simulink model "model"  (Simulink 8.7)
settings: Solver=VariableStepAuto  SolverMode=SingleTasking  StartTime=0.0  StopTime=10.0  RelTol=1e-3
settings Model: Creator=Kostyaj  LastModifiedBy=morozov
settings DataIOCC: LimitDataPoints=off  SaveFormat=Dataset
settings DebuggingCC: UnderspecifiedInitializationDetection=Simplified  MergeDetectMultiDrivingBlocksExec=error  SFUnexpectedBacktrackingDiag=error  SFNoUnconditionalDefaultTransitionDiag=error
settings HardwareCC: ProdBitPerPointer=64  ProdLargestAtomicFloat=Float  ProdIntDivRoundTo=Zero  ProdEndianess=LittleEndian  ProdWordSize=64  ProdHWDeviceType=Intel->x86-64 (Windows64)
settings ModelReferenceCC: PropagateSignalLabelsOutOfModel=on
settings GRTTargetCC: TargetLangStandard=C99 (ISO)  GeneratePreprocessorConditionals=Use local settings
settings ConfigComp: CovMetricSettings=dwe  CovHtmlReporting=off  CovSaveCumulativeToWorkspaceVar=off  CovSaveSingleToWorkspaceVar=off  CovModelRefEnable=off  CovExternalEMLEnable=on

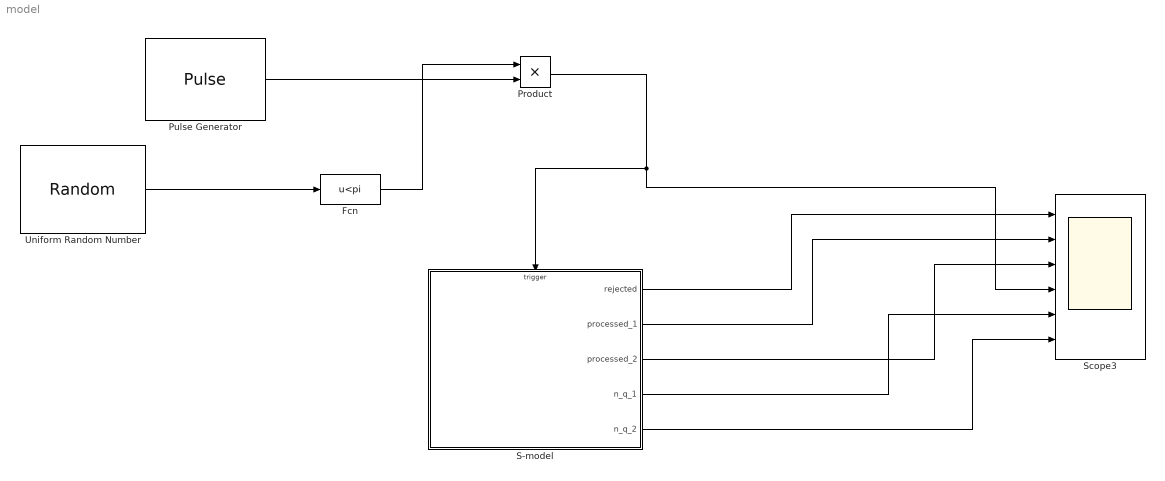
== system model ==
  Fcn : Fcn  Expr=u<pi
  Product : Product
  Pulse Generator : DiscretePulseGenerator  PulseType=Time based  Period=10  PulseWidth=5
  "S-model " : Stateflow chart  TreatAsAtomicUnit=on
  Scope3 : Scope  NumInputPorts=6
  Uniform Random Number : UniformRandomNumber  SampleTime=0.1
  wires:
  Uniform Random Number/1 -> Fcn/1
  Fcn/1 -> Product/1
  Pulse Generator/1 -> Product/2
  Product/1 -> "S-model "/Trigger, Scope3/4
  "S-model "/1(rejected) -> Scope3/1
  "S-model "/2(processed_1) -> Scope3/2
  "S-model "/3(processed_2) -> Scope3/3
  "S-model "/4(n_q_1) -> Scope3/5
  "S-model "/5(n_q_2) -> Scope3/6

== stateflow chart S-model  ==
  settings: sampleTime=Ts
  state Generator [parallel]
    settings: executionOrder=1
    state free/
    (junction 23) -> Generator.free [order 2] : [in(Q1.Process.free)]
        | {send(query, Q1.Process);}
    (junction 23) -> Generator.free [order 1] : [in(Q1.Process.busy)]
        | {send(query, Q1.Queue);}
    (junction 25) -> (junction 23) [order 1] : [n_q_1 <= n_q_2 && n_q_1 ~= ml.n_q_m]
    (junction 24) -> Generator.free [order 2] : [in(Q2.Process.busy)]
        | {send(query, Q2.Queue);}
    (junction 24) -> Generator.free [order 1] : [in(Q2.Process.free)]
        | {send(query, Q2.Process);}
    (junction 25) -> Generator.free [order 3] : [n_q_1 == ml.n_q_m && n_q_2 == ml.n_q_m]
        | {rejected = 1;}
    Generator.free -> (junction 25) : init {generated = 1;
        | n_g++; ml.n_generated = n_g;
        | ml.t_0[n_g] = t;}
    (junction 25) -> (junction 24) [order 2] : [n_q_2 < n_q_1]
  state Q2 [parallel]
    settings: executionOrder=3
    state Process [parallel]
      settings: executionOrder=1
      state busy/
        entry: t_o = t; t_mu = ml('pro(mu/2)');
        during: processed_2 = 0;
      state free/
        during: processed_2 = 0;
      Q2.Process.free -> Q2.Process.busy : query{no = n_g;}
      Q2.Process.busy -> (junction 37) : [t - t_o >= t_mu] {processed_2 = 1;}
      (junction 37) -> Q2.Process.busy [order 1] : [n_q_2 > 0] {no = ml.n_next_2[1];
          | ml.t_1[no] = t - ml.t_0[no];
          | n_p++; ml.n_queued = n_p;
          | send(prf, Q2.Queue);}
      (junction 37) -> Q2.Process.free [order 2]
      (default) -> Q2.Process.free
    state Queue [parallel]
      settings: executionOrder=2
      state empty/
      state stored/
        on query:n_q_2++;
        ml.n_next_2[n_q_2] = n_g;
        on prf: n_q_2--;
        ml.tmp = n_q_2;
        ml('n_next_2 = shif(n_next_2, tmp);');
      state full/
        exit: n_q_2--;
        ml.tmp = n_q_2;
        ml('n_next_2 = shif(n_next_2, tmp);');
      (default) -> Q2.Queue.empty
      Q2.Queue.empty -> Q2.Queue.stored : query{n_q_2++;
          | ml.n_next_2[n_q_2] = n_g;}
      Q2.Queue.stored -> Q2.Queue.empty [order 2] : [n_q_2 == 0]
      Q2.Queue.full -> Q2.Queue.stored : prf
      Q2.Queue.stored -> Q2.Queue.full [order 1] : [n_q_2 > ml.n_q_m - 1]
  state Q1 [parallel]
    settings: executionOrder=2
    state Process [parallel]
      settings: executionOrder=1
      state busy/
        entry: t_o = t; t_mu = ml('pro(mu)');
        during: processed_1 = 0;
      state free/
        during: processed_1 = 0;
      Q1.Process.free -> Q1.Process.busy : query{no = n_g;}
      Q1.Process.busy -> (junction 51) : [t - t_o >= t_mu] {processed_1 = 1;}
      (junction 51) -> Q1.Process.busy [order 1] : [n_q_1 > 0] {no = ml.n_next_1[1];
          | ml.t_1[no] = t - ml.t_0[no];
          | n_p++; ml.n_queued = n_p;
          | send(prf, Q1.Queue);}
      (junction 51) -> Q1.Process.free [order 2]
      (default) -> Q1.Process.free
    state Queue [parallel]
      settings: executionOrder=2
      state empty/
      state stored/
        on query:n_q_1++;
        ml.n_next_1[n_q_1] = n_g;
        on prf: n_q_1--;
        ml.tmp = n_q_1;
        ml('n_next_1 = shif(n_next_1, tmp);');
      state full/
        exit: n_q_1--;
        ml.tmp = n_q_1;
        ml('n_next_1 = shif(n_next_1, tmp);');
      (default) -> Q1.Queue.empty
      Q1.Queue.empty -> Q1.Queue.stored : query{n_q_1++;
          | ml.n_next_1[n_q_1] = n_g;}
      Q1.Queue.stored -> Q1.Queue.empty [order 2] : [n_q_1 == 0]
      Q1.Queue.full -> Q1.Queue.stored : prf
      Q1.Queue.stored -> Q1.Queue.full [order 1] : [n_q_1 > ml.n_q_m - 1]
  data: t_a local double; t_lambda local double; t_o local double; t_mu local double; t_o local double; t_mu local double; n_g local double; rejected output double; processed_1 output double; processed_2 output double; n_p local double; no local double; n_q_1 output double; n_q_2 output double
  events: prf local FUNCTION_CALL_EVENT; prf local FUNCTION_CALL_EVENT; query local FUNCTION_CALL_EVENT; init input FALLING_EDGE_EVENT
